simulink model "discrete_model"  (R2020a)
settings: Solver=ode45  StartTime=0.0  StopTime=10.0  RelTol=1e-3
undefined symbols (not defined in the file): DiscIntNeverNeededParam
settings Model: Creator=11973  LastModifiedBy=11973

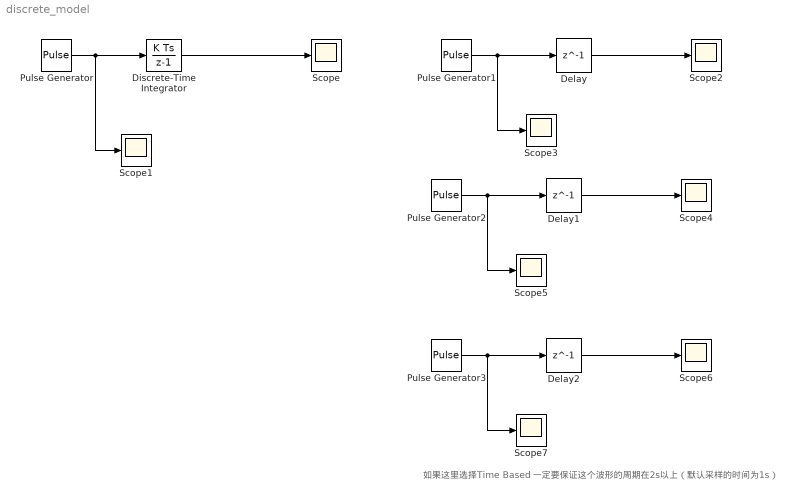
== system discrete_model ==
  note: 如果这里选择Time Based 一定要保证这个波形的周期在2s以上（默认采样的时间为1s）
  Delay : Delay  DelayLength=1  InitialCondition=0
  Delay1 : Delay  DelayLength=1  InitialCondition=0
  Delay2 : Delay  DelayLength=1  InitialCondition=0
  Discrete-Time Integrator : DiscreteIntegrator  SampleTime=-1  ICPrevOutput=DiscIntNeverNeededParam  ICPrevScaledInput=DiscIntNeverNeededParam
  Pulse Generator : DiscretePulseGenerator  PulseType=Time based  PulseWidth=50
  Pulse Generator1 : DiscretePulseGenerator
  Pulse Generator2 : DiscretePulseGenerator  PulseType=Time based  PulseWidth=50
  Pulse Generator3 : DiscretePulseGenerator  PulseType=Time based  Period=4  PulseWidth=50
  Scope{,1..7} (8 alike) : Scope
  wires:
  Pulse Generator/1 -> Scope1/1, Discrete-Time Integrator/1
  Discrete-Time Integrator/1 -> Scope/1
  Pulse Generator1/1 -> Scope3/1, Delay/1
  Delay/1 -> Scope2/1
  Delay1/1 -> Scope4/1
  Pulse Generator2/1 -> Delay1/1, Scope5/1
  Pulse Generator3/1 -> Scope7/1, Delay2/1
  Delay2/1 -> Scope6/1
